simulink model "SteeringWheel"  (R2024b)
settings: configuration reference "STM32H7_Config" (kept outside this file)
settings Model: DataDictionary=Master_Dictionary.sldd  EnableAccessToBaseWorkspace=off  Creator=torni  LastModifiedBy=William
settings ConfigSetRef: SourceName=STM32H7_Config

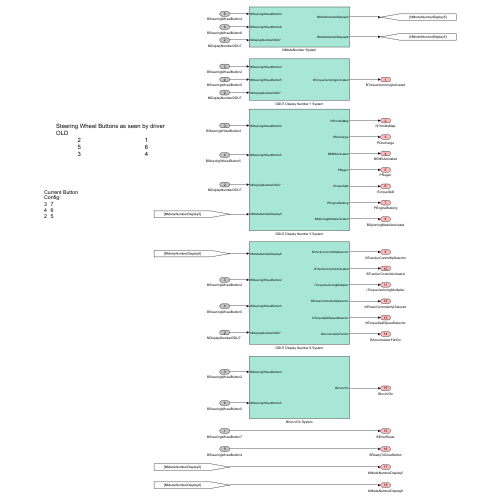
[thumbnail: Simulink's stored preview of the top-level diagram]
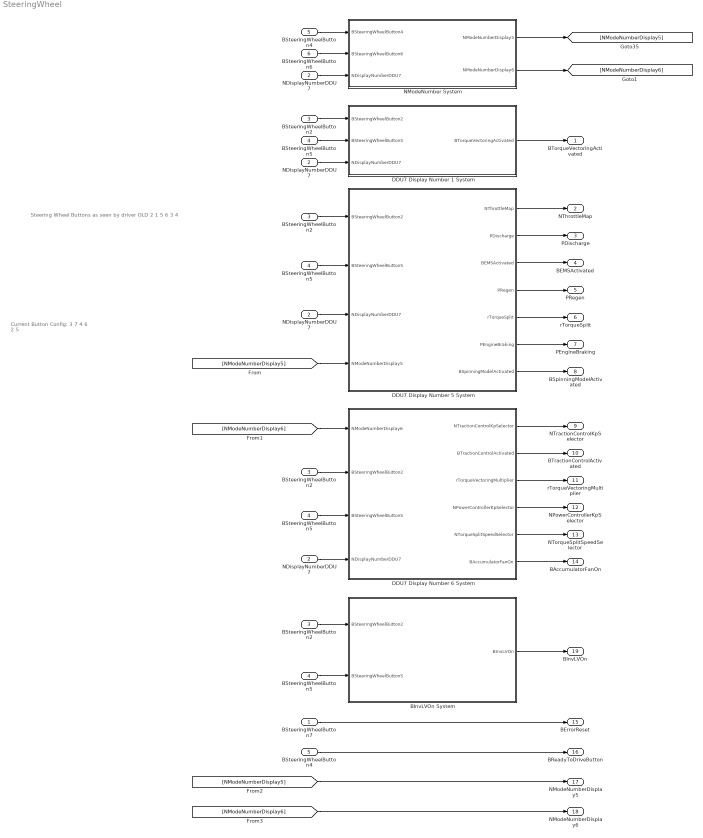
== system SteeringWheel ==
  note: Current Button Config:
      | 3 7
      | 4 6
      | 2 5
  note: Steering Wheel Buttons as seen by driver
      | OLD
      | 2 1
      | 5 6
      | 3 4
  BSteeringWheelButton7 : Inport  OutDataTypeStr=boolean
  NDisplayNumberDDU7 : Inport  Port=2  OutDataTypeStr=double
  "BSteeringWheelButton2 " : Inport  Port=3  OutDataTypeStr=boolean
  "BSteeringWheelButton5 " : Inport  Port=4  OutDataTypeStr=boolean
  BSteeringWheelButton4 : Inport  Port=5  OutDataTypeStr=boolean
  BSteeringWheelButton6 : Inport  Port=6  OutDataTypeStr=boolean
  BInvLVOn System : Subsystem
  "BSteeringWheelButton2 " : InportShadow  Port=3  OutDataTypeStr=boolean
  "BSteeringWheelButton2 " : InportShadow  Port=3  OutDataTypeStr=boolean
  "BSteeringWheelButton2  " : InportShadow  Port=3  OutDataTypeStr=boolean
  "BSteeringWheelButton4 " : InportShadow  Port=5  OutDataTypeStr=boolean
  "BSteeringWheelButton5 " : InportShadow  Port=4  OutDataTypeStr=boolean
  "BSteeringWheelButton5 " : InportShadow  Port=4  OutDataTypeStr=boolean
  "BSteeringWheelButton5   " : InportShadow  Port=4  OutDataTypeStr=boolean
  DDU7 Display Number 1 System : Subsystem
  DDU7 Display Number 5 System : Subsystem
  DDU7 Display Number 6 System : Subsystem
  "NDisplayNumberDDU7 " : InportShadow  Port=2  OutDataTypeStr=double
  "NDisplayNumberDDU7 " : InportShadow  Port=2  OutDataTypeStr=double
  "NDisplayNumberDDU7  " : InportShadow  Port=2  OutDataTypeStr=double
  NModeNumber System : Subsystem
  BTorqueVectoringActivated : Outport  OutDataTypeStr=boolean  VectorParamsAs1DForOutWhenUnconnected=off
  NThrottleMap : Outport  Port=2  OutDataTypeStr=double  VectorParamsAs1DForOutWhenUnconnected=off
  PDischarge : Outport  Port=3  OutDataTypeStr=double  VectorParamsAs1DForOutWhenUnconnected=off
  BEMSActivated : Outport  Port=4  OutDataTypeStr=boolean  VectorParamsAs1DForOutWhenUnconnected=off
  PRegen : Outport  Port=5  OutDataTypeStr=double  VectorParamsAs1DForOutWhenUnconnected=off
  rTorqueSplit : Outport  Port=6  OutDataTypeStr=double  VectorParamsAs1DForOutWhenUnconnected=off
  PEngineBraking : Outport  Port=7  OutDataTypeStr=double  VectorParamsAs1DForOutWhenUnconnected=off
  BSpinningModelActivated : Outport  Port=8  OutDataTypeStr=boolean  VectorParamsAs1DForOutWhenUnconnected=off
  NTractionControlKpSelector : Outport  Port=9  OutDataTypeStr=double  VectorParamsAs1DForOutWhenUnconnected=off
  BTractionControlActivated : Outport  Port=10  OutDataTypeStr=boolean  VectorParamsAs1DForOutWhenUnconnected=off
  rTorqueVectoringMultiplier : Outport  Port=11  OutDataTypeStr=double  VectorParamsAs1DForOutWhenUnconnected=off
  NPowerControllerKpSelector : Outport  Port=12  OutDataTypeStr=double  VectorParamsAs1DForOutWhenUnconnected=off
  NTorqueSplitSpeedSelector : Outport  Port=13  OutDataTypeStr=double  VectorParamsAs1DForOutWhenUnconnected=off
  BAccumulatorFanOn : Outport  Port=14  OutDataTypeStr=boolean  VectorParamsAs1DForOutWhenUnconnected=off
  BErrorReset : Outport  Port=15  OutDataTypeStr=boolean  VectorParamsAs1DForOutWhenUnconnected=off
  BReadyToDriveButton : Outport  Port=16  OutDataTypeStr=boolean  VectorParamsAs1DForOutWhenUnconnected=off
  NModeNumberDisplay5 : Outport  Port=17  OutDataTypeStr=double  VectorParamsAs1DForOutWhenUnconnected=off
  NModeNumberDisplay6 : Outport  Port=18  OutDataTypeStr=double  VectorParamsAs1DForOutWhenUnconnected=off
  BInvLVOn : Outport  Port=19  OutDataTypeStr=boolean  VectorParamsAs1DForOutWhenUnconnected=off
  wires:
  "BSteeringWheelButton5 "/1 -> DDU7 Display Number 1 System/2("BSteeringWheelButton5 ")
  "BSteeringWheelButton2 "/1 -> DDU7 Display Number 1 System/1("BSteeringWheelButton2 ")
  NDisplayNumberDDU7/1 -> DDU7 Display Number 1 System/3(NDisplayNumberDDU7)
  "NDisplayNumberDDU7 "/1 -> DDU7 Display Number 5 System/3(NDisplayNumberDDU7)
  "NDisplayNumberDDU7  "/1 -> DDU7 Display Number 6 System/4("NDisplayNumberDDU7  ")
  NModeNumber System/1(NModeNumberDisplay5) -> [NModeNumberDisplay5]
  NModeNumber System/2(NModeNumberDisplay6) -> [NModeNumberDisplay6]
  "BSteeringWheelButton2  "/1 -> DDU7 Display Number 5 System/1("BSteeringWheelButton2  ")
  "BSteeringWheelButton5   "/1 -> DDU7 Display Number 5 System/2("BSteeringWheelButton5  ")
  "BSteeringWheelButton2 "/1 -> DDU7 Display Number 6 System/2("BSteeringWheelButton2 ")
  "BSteeringWheelButton5 "/1 -> DDU7 Display Number 6 System/3("BSteeringWheelButton5 ")
  DDU7 Display Number 5 System/6(PEngineBraking) -> PEngineBraking/1
  DDU7 Display Number 5 System/1(NThrottleMap) -> NThrottleMap/1
  DDU7 Display Number 5 System/5(rTorqueSplit) -> rTorqueSplit/1
  DDU7 Display Number 5 System/4(PRegen) -> PRegen/1
  DDU7 Display Number 6 System/1(NTractionControlKpSelector) -> NTractionControlKpSelector/1
  DDU7 Display Number 6 System/3(rTorqueVectoringMultiplier) -> rTorqueVectoringMultiplier/1
  DDU7 Display Number 6 System/4(NPowerControllerKpSelector) -> NPowerControllerKpSelector/1
  DDU7 Display Number 6 System/5(NTorqueSplitSpeedSelector) -> NTorqueSplitSpeedSelector/1
  BSteeringWheelButton7/1 -> BErrorReset/1
  "NDisplayNumberDDU7 "/1 -> NModeNumber System/3("NDisplayNumberDDU7 ")
  BSteeringWheelButton4/1 -> NModeNumber System/1("BSteeringWheelButton4 ")
  BSteeringWheelButton6/1 -> NModeNumber System/2("BSteeringWheelButton6 ")
  DDU7 Display Number 5 System/2(PDischarge) -> PDischarge/1
  "BSteeringWheelButton4 "/1 -> BReadyToDriveButton/1
  [NModeNumberDisplay5] -> DDU7 Display Number 5 System/4(NModeNumberDisplay5)
  [NModeNumberDisplay6] -> DDU7 Display Number 6 System/1(NModeNumberDisplay6)
  [NModeNumberDisplay5] -> NModeNumberDisplay5/1
  [NModeNumberDisplay6] -> NModeNumberDisplay6/1
  DDU7 Display Number 6 System/6(BAccumulatorFanOn) -> BAccumulatorFanOn/1
  DDU7 Display Number 6 System/2(BTractionControlActivated) -> BTractionControlActivated/1
  DDU7 Display Number 5 System/7(BSpinningModelActivated) -> BSpinningModelActivated/1
  DDU7 Display Number 5 System/3(BEMSActivated) -> BEMSActivated/1
  DDU7 Display Number 1 System/1(BTorqueVectoringActivated) -> BTorqueVectoringActivated/1
  "BSteeringWheelButton5 "/1 -> BInvLVOn System/2(BSteeringWheelButton5)
  "BSteeringWheelButton2 "/1 -> BInvLVOn System/1("BSteeringWheelButton2 ")
  BInvLVOn System/1(BInvLVOn) -> BInvLVOn/1

== system SteeringWheel/BInvLVOn System ==
  "BSteeringWheelButton2 " : Inport  OutDataTypeStr=boolean
  BSteeringWheelButton5 : Inport  Port=2  OutDataTypeStr=boolean
  AND : Logic  Operator=NAND  AllPortsSameDT=off  OutDataTypeStr=boolean
  BInvLVOn : Outport  OutDataTypeStr=boolean  VectorParamsAs1DForOutWhenUnconnected=off
  wires:
  "BSteeringWheelButton2 "/1 -> AND/1
  BSteeringWheelButton5/1 -> AND/2
  AND/1 -> BInvLVOn/1

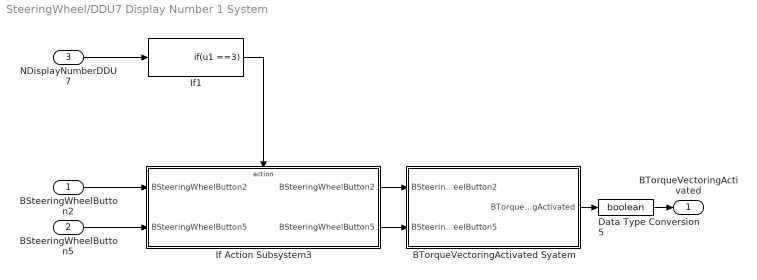
== system SteeringWheel/DDU7 Display Number 1 System ==
  "BSteeringWheelButton2 " : Inport  OutDataTypeStr=boolean
  "BSteeringWheelButton5 " : Inport  Port=2  OutDataTypeStr=boolean
  NDisplayNumberDDU7 : Inport  Port=3  OutDataTypeStr=double
  BTorqueVectoringActivated Syatem : Stateflow chart  TreatAsAtomicUnit=on
  Data Type Conversion5 : DataTypeConversion  OutDataTypeStr=boolean  SaturateOnIntegerOverflow=off  RndMeth=Floor
  If Action Subsystem3 : Subsystem  TreatAsAtomicUnit=on
  If1 : If  IfExpression=u1 ==3  ShowElse=off
  BTorqueVectoringActivated : Outport  OutDataTypeStr=boolean  VectorParamsAs1DForOutWhenUnconnected=off
  wires:
  If Action Subsystem3/1(BSteeringWheelButton2) -> BTorqueVectoringActivated Syatem/1(BSteeringWheelButton2)
  If Action Subsystem3/2(BSteeringWheelButton5) -> BTorqueVectoringActivated Syatem/2(BSteeringWheelButton5)
  If1/1 -> If Action Subsystem3/Action
  NDisplayNumberDDU7/1 -> If1/1
  "BSteeringWheelButton2 "/1 -> If Action Subsystem3/1("BSteeringWheelButton2 ")
  "BSteeringWheelButton5 "/1 -> If Action Subsystem3/2("BSteeringWheelButton5 ")
  Data Type Conversion5/1 -> BTorqueVectoringActivated/1
  BTorqueVectoringActivated Syatem/1(BTorqueVectoringActivated) -> Data Type Conversion5/1

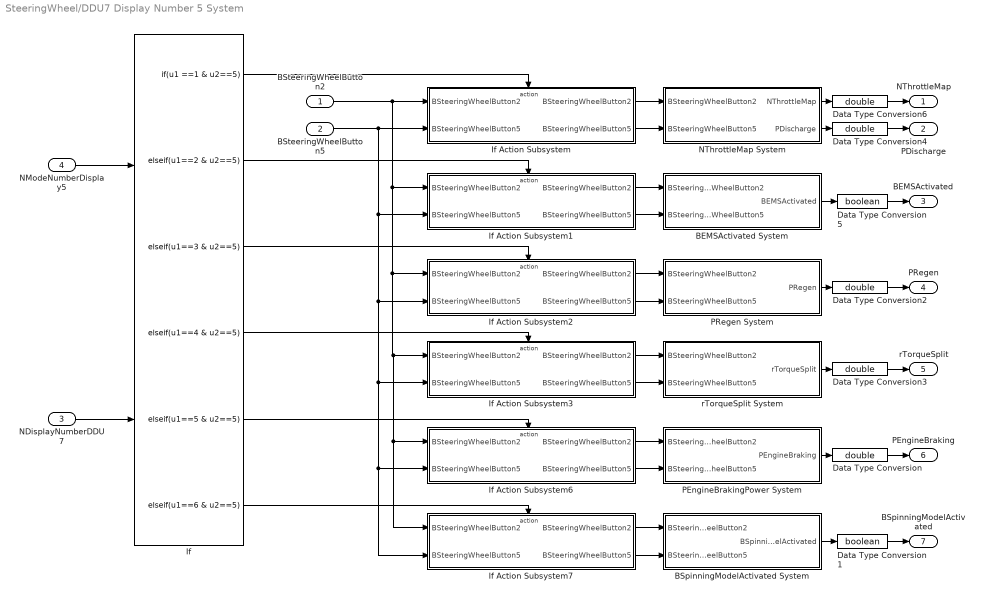
== system SteeringWheel/DDU7 Display Number 5 System ==
  "BSteeringWheelButton2  " : Inport  OutDataTypeStr=boolean
  "BSteeringWheelButton5  " : Inport  Port=2  OutDataTypeStr=boolean
  NDisplayNumberDDU7 : Inport  Port=3  OutDataTypeStr=double
  NModeNumberDisplay5 : Inport  Port=4  OutDataTypeStr=double
  BEMSActivated System : Stateflow chart  TreatAsAtomicUnit=on
  BSpinningModelActivated System : Stateflow chart  TreatAsAtomicUnit=on
  Data Type Conversion{,2..4,6} (5 alike) : DataTypeConversion  OutDataTypeStr=double  SaturateOnIntegerOverflow=off  RndMeth=Floor
  Data Type Conversion1 : DataTypeConversion  OutDataTypeStr=boolean  SaturateOnIntegerOverflow=off  RndMeth=Floor
  Data Type Conversion5 : DataTypeConversion  OutDataTypeStr=boolean  SaturateOnIntegerOverflow=off  RndMeth=Floor
  If : If  NumInputs=2  IfExpression=u1 ==1 & u2==5  ElseIfExpressions=u1==2 & u2==5,u1==3 & u2==5,u1==4 & u2==5 ,u1==5 & u2==5,u1==6 & u2==5  ShowElse=off
  If Action Subsystem : Subsystem  TreatAsAtomicUnit=on
  If Action Subsystem1 : Subsystem  TreatAsAtomicUnit=on
  If Action Subsystem2 : Subsystem  TreatAsAtomicUnit=on
  If Action Subsystem3 : Subsystem  TreatAsAtomicUnit=on
  If Action Subsystem6 : Subsystem  TreatAsAtomicUnit=on
  If Action Subsystem7 : Subsystem  TreatAsAtomicUnit=on
  NThrottleMap System : Stateflow chart  TreatAsAtomicUnit=on
  PEngineBrakingPower System : Stateflow chart  TreatAsAtomicUnit=on
  PRegen System : Stateflow chart  TreatAsAtomicUnit=on
  rTorqueSplit System : Stateflow chart  TreatAsAtomicUnit=on
  NThrottleMap : Outport  OutDataTypeStr=double  VectorParamsAs1DForOutWhenUnconnected=off
  PDischarge : Outport  Port=2  OutDataTypeStr=double  VectorParamsAs1DForOutWhenUnconnected=off
  BEMSActivated : Outport  Port=3  OutDataTypeStr=boolean  VectorParamsAs1DForOutWhenUnconnected=off
  PRegen : Outport  Port=4  OutDataTypeStr=double  VectorParamsAs1DForOutWhenUnconnected=off
  rTorqueSplit : Outport  Port=5  OutDataTypeStr=double  VectorParamsAs1DForOutWhenUnconnected=off
  PEngineBraking : Outport  Port=6  OutDataTypeStr=double  VectorParamsAs1DForOutWhenUnconnected=off
  BSpinningModelActivated : Outport  Port=7  OutDataTypeStr=boolean  VectorParamsAs1DForOutWhenUnconnected=off
  wires:
  NModeNumberDisplay5/1 -> If/1
  If Action Subsystem/2(BSteeringWheelButton5) -> NThrottleMap System/2(BSteeringWheelButton5)
  If Action Subsystem/1(BSteeringWheelButton2) -> NThrottleMap System/1(BSteeringWheelButton2)
  NThrottleMap System/1(NThrottleMap) -> Data Type Conversion6/1
  BEMSActivated System/1(BEMSActivated) -> Data Type Conversion5/1
  If Action Subsystem2/1(BSteeringWheelButton2) -> PRegen System/1(BSteeringWheelButton2)
  If Action Subsystem2/2(BSteeringWheelButton5) -> PRegen System/2(BSteeringWheelButton5)
  PRegen System/1(PRegen) -> Data Type Conversion2/1
  If Action Subsystem3/1(BSteeringWheelButton2) -> rTorqueSplit System/1(BSteeringWheelButton2)
  If Action Subsystem3/2(BSteeringWheelButton5) -> rTorqueSplit System/2(BSteeringWheelButton5)
  rTorqueSplit System/1(rTorqueSplit) -> Data Type Conversion3/1
  If Action Subsystem6/2(BSteeringWheelButton5) -> PEngineBrakingPower System/2(BSteeringWheelButton5)
  PEngineBrakingPower System/1(PEngineBraking) -> Data Type Conversion/1
  If Action Subsystem6/1(BSteeringWheelButton2) -> PEngineBrakingPower System/1(BSteeringWheelButton2)
  If Action Subsystem7/2(BSteeringWheelButton5) -> BSpinningModelActivated System/2(BSteeringWheelButton5)
  BSpinningModelActivated System/1(BSpinningModelActivated) -> Data Type Conversion1/1
  If Action Subsystem7/1(BSteeringWheelButton2) -> BSpinningModelActivated System/1(BSteeringWheelButton2)
  If/4 -> If Action Subsystem3/Action
  If/3 -> If Action Subsystem2/Action
  If/2 -> If Action Subsystem1/Action
  If/1 -> If Action Subsystem/Action
  If/5 -> If Action Subsystem6/Action
  If/6 -> If Action Subsystem7/Action
  NDisplayNumberDDU7/1 -> If/2
  "BSteeringWheelButton5  "/1 -> If Action Subsystem6/2("BSteeringWheelButton5  "), If Action Subsystem7/2("BSteeringWheelButton5  "), If Action Subsystem3/2("BSteeringWheelButton5  "), If Action Subsystem2/2("BSteeringWheelButton5  "), If Action Subsystem1/2("BSteeringWheelButton5  "), If Action Subsystem/2("BSteeringWheelButton5  ")
  "BSteeringWheelButton2  "/1 -> If Action Subsystem6/1("BSteeringWheelButton2  "), If Action Subsystem7/1("BSteeringWheelButton2  "), If Action Subsystem3/1("BSteeringWheelButton2  "), If Action Subsystem2/1("BSteeringWheelButton2  "), If Action Subsystem1/1("BSteeringWheelButton2  "), If Action Subsystem/1("BSteeringWheelButton2  ")
  If Action Subsystem1/1(BSteeringWheelButton2) -> BEMSActivated System/1(BSteeringWheelButton2)
  If Action Subsystem1/2(BSteeringWheelButton5) -> BEMSActivated System/2(BSteeringWheelButton5)
  NThrottleMap System/2(PDischarge) -> Data Type Conversion4/1
  Data Type Conversion5/1 -> BEMSActivated/1
  Data Type Conversion1/1 -> BSpinningModelActivated/1
  Data Type Conversion/1 -> PEngineBraking/1
  Data Type Conversion2/1 -> PRegen/1
  Data Type Conversion3/1 -> rTorqueSplit/1
  Data Type Conversion4/1 -> PDischarge/1
  Data Type Conversion6/1 -> NThrottleMap/1

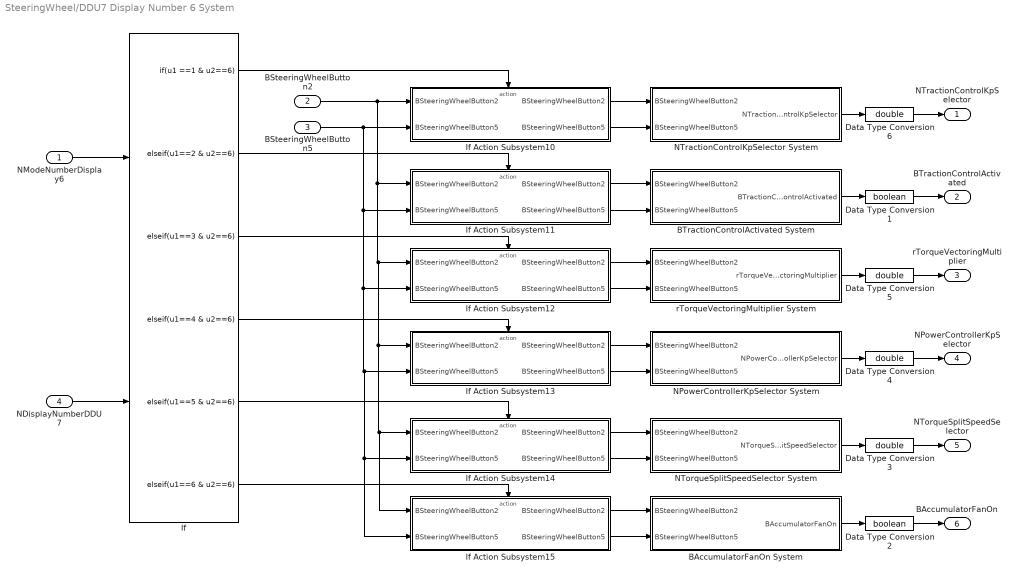
== system SteeringWheel/DDU7 Display Number 6 System ==
  NModeNumberDisplay6 : Inport  OutDataTypeStr=double
  "BSteeringWheelButton2 " : Inport  Port=2  OutDataTypeStr=boolean
  "BSteeringWheelButton5 " : Inport  Port=3  OutDataTypeStr=boolean
  "NDisplayNumberDDU7  " : Inport  Port=4  OutDataTypeStr=double
  BAccumulatorFanOn System : Stateflow chart  TreatAsAtomicUnit=on
  BTractionControlActivated System : Stateflow chart  TreatAsAtomicUnit=on
  Data Type Conversion1 : DataTypeConversion  OutDataTypeStr=boolean  SaturateOnIntegerOverflow=off  RndMeth=Floor
  Data Type Conversion2 : DataTypeConversion  OutDataTypeStr=boolean  SaturateOnIntegerOverflow=off  RndMeth=Floor
  Data Type Conversion{3..6} (4 alike) : DataTypeConversion  OutDataTypeStr=double  SaturateOnIntegerOverflow=off  RndMeth=Floor
  If : If  NumInputs=2  IfExpression=u1 ==1 & u2==6  ElseIfExpressions=u1==2 & u2==6,u1==3 & u2==6,u1==4 & u2==6,u1==5 & u2==6,u1==6 & u2==6  ShowElse=off
  If Action Subsystem10 : Subsystem  TreatAsAtomicUnit=on
  If Action Subsystem11 : Subsystem  TreatAsAtomicUnit=on
  If Action Subsystem12 : Subsystem  TreatAsAtomicUnit=on
  If Action Subsystem13 : Subsystem  TreatAsAtomicUnit=on
  If Action Subsystem14 : Subsystem  TreatAsAtomicUnit=on
  If Action Subsystem15 : Subsystem  TreatAsAtomicUnit=on
  NPowerControllerKpSelector System : Stateflow chart  TreatAsAtomicUnit=on
  NTorqueSplitSpeedSelector System : Stateflow chart  TreatAsAtomicUnit=on
  NTractionControlKpSelector System : Stateflow chart  TreatAsAtomicUnit=on
  rTorqueVectoringMultiplier System : Stateflow chart  TreatAsAtomicUnit=on
  NTractionControlKpSelector : Outport  OutDataTypeStr=double  VectorParamsAs1DForOutWhenUnconnected=off
  BTractionControlActivated : Outport  Port=2  OutDataTypeStr=boolean  VectorParamsAs1DForOutWhenUnconnected=off
  rTorqueVectoringMultiplier : Outport  Port=3  OutDataTypeStr=double  VectorParamsAs1DForOutWhenUnconnected=off
  NPowerControllerKpSelector : Outport  Port=4  OutDataTypeStr=double  VectorParamsAs1DForOutWhenUnconnected=off
  NTorqueSplitSpeedSelector : Outport  Port=5  OutDataTypeStr=double  VectorParamsAs1DForOutWhenUnconnected=off
  BAccumulatorFanOn : Outport  Port=6  OutDataTypeStr=boolean  VectorParamsAs1DForOutWhenUnconnected=off
  wires:
  If Action Subsystem15/1(BSteeringWheelButton2) -> BAccumulatorFanOn System/1(BSteeringWheelButton2)
  BAccumulatorFanOn System/1(BAccumulatorFanOn) -> Data Type Conversion2/1
  If Action Subsystem15/2(BSteeringWheelButton5) -> BAccumulatorFanOn System/2(BSteeringWheelButton5)
  If Action Subsystem14/1(BSteeringWheelButton2) -> NTorqueSplitSpeedSelector System/1(BSteeringWheelButton2)
  NTorqueSplitSpeedSelector System/1(NTorqueSplitSpeedSelector) -> Data Type Conversion3/1
  If Action Subsystem14/2(BSteeringWheelButton5) -> NTorqueSplitSpeedSelector System/2(BSteeringWheelButton5)
  If Action Subsystem13/2(BSteeringWheelButton5) -> NPowerControllerKpSelector System/2(BSteeringWheelButton5)
  If Action Subsystem13/1(BSteeringWheelButton2) -> NPowerControllerKpSelector System/1(BSteeringWheelButton2)
  NPowerControllerKpSelector System/1(NPowerControllerKpSelector) -> Data Type Conversion4/1
  rTorqueVectoringMultiplier System/1(rTorqueVectoringMultiplier) -> Data Type Conversion5/1
  If Action Subsystem12/2(BSteeringWheelButton5) -> rTorqueVectoringMultiplier System/2(BSteeringWheelButton5)
  If Action Subsystem12/1(BSteeringWheelButton2) -> rTorqueVectoringMultiplier System/1(BSteeringWheelButton2)
  BTractionControlActivated System/1(BTractionControlActivated) -> Data Type Conversion1/1
  If Action Subsystem11/2(BSteeringWheelButton5) -> BTractionControlActivated System/2(BSteeringWheelButton5)
  If Action Subsystem11/1(BSteeringWheelButton2) -> BTractionControlActivated System/1(BSteeringWheelButton2)
  NTractionControlKpSelector System/1(NTractionControlKpSelector) -> Data Type Conversion6/1
  "BSteeringWheelButton5 "/1 -> If Action Subsystem15/2("BSteeringWheelButton5  "), If Action Subsystem14/2("BSteeringWheelButton5  "), If Action Subsystem13/2("BSteeringWheelButton5  "), If Action Subsystem12/2("BSteeringWheelButton5  "), If Action Subsystem11/2("BSteeringWheelButton5  "), If Action Subsystem10/2("BSteeringWheelButton5  ")
  If/2 -> If Action Subsystem11/Action
  If/6 -> If Action Subsystem15/Action
  If/4 -> If Action Subsystem13/Action
  If/3 -> If Action Subsystem12/Action
  If/1 -> If Action Subsystem10/Action
  "BSteeringWheelButton2 "/1 -> If Action Subsystem15/1("BSteeringWheelButton2  "), If Action Subsystem14/1("BSteeringWheelButton2  "), If Action Subsystem13/1("BSteeringWheelButton2  "), If Action Subsystem12/1("BSteeringWheelButton2  "), If Action Subsystem11/1("BSteeringWheelButton2  "), If Action Subsystem10/1("BSteeringWheelButton2  ")
  "NDisplayNumberDDU7  "/1 -> If/2
  NModeNumberDisplay6/1 -> If/1
  If/5 -> If Action Subsystem14/Action
  If Action Subsystem10/1(BSteeringWheelButton2) -> NTractionControlKpSelector System/1(BSteeringWheelButton2)
  If Action Subsystem10/2(BSteeringWheelButton5) -> NTractionControlKpSelector System/2(BSteeringWheelButton5)
  Data Type Conversion2/1 -> BAccumulatorFanOn/1
  Data Type Conversion1/1 -> BTractionControlActivated/1
  Data Type Conversion3/1 -> NTorqueSplitSpeedSelector/1
  Data Type Conversion4/1 -> NPowerControllerKpSelector/1
  Data Type Conversion5/1 -> rTorqueVectoringMultiplier/1
  Data Type Conversion6/1 -> NTractionControlKpSelector/1

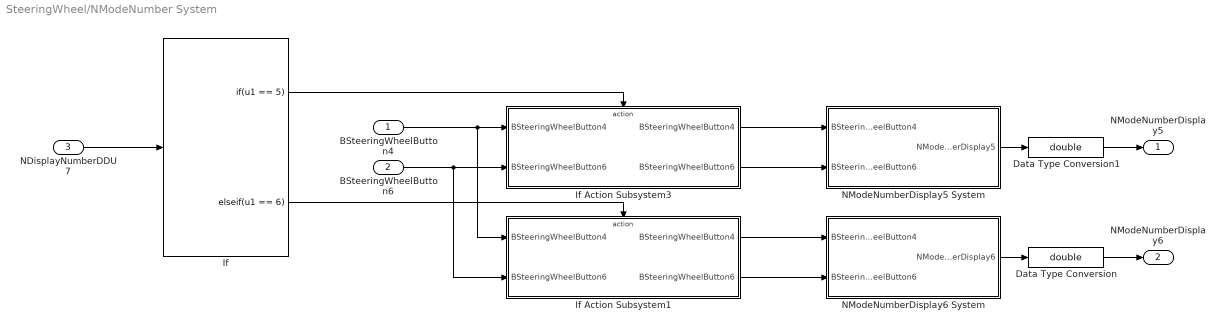
== system SteeringWheel/NModeNumber System ==
  "BSteeringWheelButton4 " : Inport  OutDataTypeStr=boolean
  "BSteeringWheelButton6 " : Inport  Port=2  OutDataTypeStr=boolean
  "NDisplayNumberDDU7 " : Inport  Port=3  OutDataTypeStr=double
  Data Type Conversion : DataTypeConversion  OutDataTypeStr=double  SaturateOnIntegerOverflow=off  RndMeth=Floor
  Data Type Conversion1 : DataTypeConversion  OutDataTypeStr=double  SaturateOnIntegerOverflow=off  RndMeth=Floor
  If : If  IfExpression=u1 == 5  ElseIfExpressions=u1 == 6  ShowElse=off
  If Action Subsystem1 : Subsystem  TreatAsAtomicUnit=on
  If Action Subsystem3 : Subsystem  TreatAsAtomicUnit=on
  NModeNumberDisplay5 System : Stateflow chart  TreatAsAtomicUnit=on
  NModeNumberDisplay6 System : Stateflow chart  TreatAsAtomicUnit=on
  NModeNumberDisplay5 : Outport  OutDataTypeStr=double  VectorParamsAs1DForOutWhenUnconnected=off
  NModeNumberDisplay6 : Outport  Port=2  OutDataTypeStr=double  VectorParamsAs1DForOutWhenUnconnected=off
  wires:
  NModeNumberDisplay5 System/1(NModeNumberDisplay5) -> Data Type Conversion1/1
  If Action Subsystem3/1(BSteeringWheelButton4) -> NModeNumberDisplay5 System/1(BSteeringWheelButton4)
  If Action Subsystem3/2(BSteeringWheelButton6) -> NModeNumberDisplay5 System/2(BSteeringWheelButton6)
  NModeNumberDisplay6 System/1(NModeNumberDisplay6) -> Data Type Conversion/1
  If Action Subsystem1/1(BSteeringWheelButton4) -> NModeNumberDisplay6 System/1(BSteeringWheelButton4)
  If Action Subsystem1/2(BSteeringWheelButton6) -> NModeNumberDisplay6 System/2(BSteeringWheelButton6)
  "NDisplayNumberDDU7 "/1 -> If/1
  "BSteeringWheelButton6 "/1 -> If Action Subsystem1/2("BSteeringWheelButton6 "), If Action Subsystem3/2("BSteeringWheelButton6 ")
  "BSteeringWheelButton4 "/1 -> If Action Subsystem1/1("BSteeringWheelButton4 "), If Action Subsystem3/1("BSteeringWheelButton4 ")
  If/1 -> If Action Subsystem3/Action
  If/2 -> If Action Subsystem1/Action
  Data Type Conversion1/1 -> NModeNumberDisplay5/1
  Data Type Conversion/1 -> NModeNumberDisplay6/1

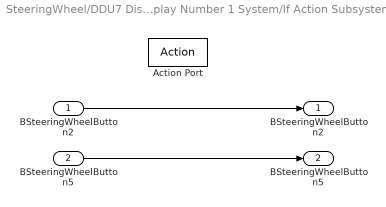
== system SteeringWheel/DDU7 Display Number 1 System/If Action Subsystem3 ==
  "BSteeringWheelButton2 " : Inport  OutDataTypeStr=boolean
  "BSteeringWheelButton5 " : Inport  Port=2  OutDataTypeStr=boolean
  Action Port : ActionPort  ActionPortLabel=if { }
  BSteeringWheelButton2 : Outport  OutDataTypeStr=boolean  VectorParamsAs1DForOutWhenUnconnected=off
  BSteeringWheelButton5 : Outport  Port=2  OutDataTypeStr=boolean  VectorParamsAs1DForOutWhenUnconnected=off
  wires:
  "BSteeringWheelButton2 "/1 -> BSteeringWheelButton2/1
  "BSteeringWheelButton5 "/1 -> BSteeringWheelButton5/1

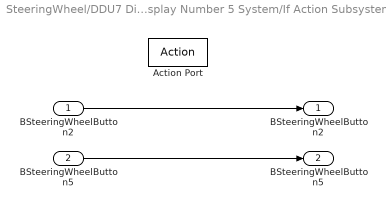
== system SteeringWheel/DDU7 Display Number 5 System/If Action Subsystem ==
  "BSteeringWheelButton2  " : Inport  OutDataTypeStr=boolean
  "BSteeringWheelButton5  " : Inport  Port=2  OutDataTypeStr=boolean
  Action Port : ActionPort  ActionPortLabel=if { }
  BSteeringWheelButton2 : Outport  OutDataTypeStr=boolean  VectorParamsAs1DForOutWhenUnconnected=off
  BSteeringWheelButton5 : Outport  Port=2  OutDataTypeStr=boolean  VectorParamsAs1DForOutWhenUnconnected=off
  wires:
  "BSteeringWheelButton2  "/1 -> BSteeringWheelButton2/1
  "BSteeringWheelButton5  "/1 -> BSteeringWheelButton5/1

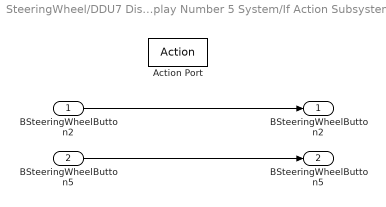
== system SteeringWheel/DDU7 Display Number 5 System/If Action Subsystem1 ==
  "BSteeringWheelButton2  " : Inport  OutDataTypeStr=boolean
  "BSteeringWheelButton5  " : Inport  Port=2  OutDataTypeStr=boolean
  Action Port : ActionPort  ActionPortLabel=elseif { }
  BSteeringWheelButton2 : Outport  OutDataTypeStr=boolean  VectorParamsAs1DForOutWhenUnconnected=off
  BSteeringWheelButton5 : Outport  Port=2  OutDataTypeStr=boolean  VectorParamsAs1DForOutWhenUnconnected=off
  wires:
  "BSteeringWheelButton5  "/1 -> BSteeringWheelButton5/1
  "BSteeringWheelButton2  "/1 -> BSteeringWheelButton2/1

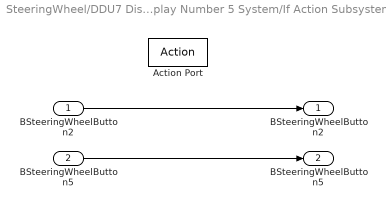
== system SteeringWheel/DDU7 Display Number 5 System/If Action Subsystem2 ==
  "BSteeringWheelButton2  " : Inport  OutDataTypeStr=boolean
  "BSteeringWheelButton5  " : Inport  Port=2  OutDataTypeStr=boolean
  Action Port : ActionPort  ActionPortLabel=elseif { }
  BSteeringWheelButton2 : Outport  OutDataTypeStr=boolean  VectorParamsAs1DForOutWhenUnconnected=off
  BSteeringWheelButton5 : Outport  Port=2  OutDataTypeStr=boolean  VectorParamsAs1DForOutWhenUnconnected=off
  wires:
  "BSteeringWheelButton2  "/1 -> BSteeringWheelButton2/1
  "BSteeringWheelButton5  "/1 -> BSteeringWheelButton5/1

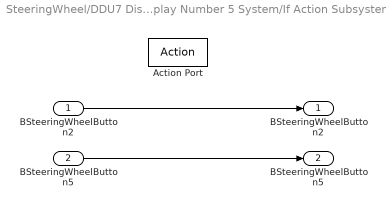
== system SteeringWheel/DDU7 Display Number 5 System/If Action Subsystem3 ==
  "BSteeringWheelButton2  " : Inport  OutDataTypeStr=boolean
  "BSteeringWheelButton5  " : Inport  Port=2  OutDataTypeStr=boolean
  Action Port : ActionPort  ActionPortLabel=elseif { }
  BSteeringWheelButton2 : Outport  OutDataTypeStr=boolean  VectorParamsAs1DForOutWhenUnconnected=off
  BSteeringWheelButton5 : Outport  Port=2  OutDataTypeStr=boolean  VectorParamsAs1DForOutWhenUnconnected=off
  wires:
  "BSteeringWheelButton5  "/1 -> BSteeringWheelButton5/1
  "BSteeringWheelButton2  "/1 -> BSteeringWheelButton2/1

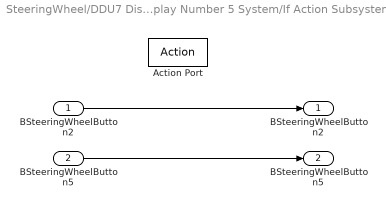
== system SteeringWheel/DDU7 Display Number 5 System/If Action Subsystem6 ==
  "BSteeringWheelButton2  " : Inport  OutDataTypeStr=boolean
  "BSteeringWheelButton5  " : Inport  Port=2  OutDataTypeStr=boolean
  Action Port : ActionPort  ActionPortLabel=elseif { }
  BSteeringWheelButton2 : Outport  OutDataTypeStr=boolean  VectorParamsAs1DForOutWhenUnconnected=off
  BSteeringWheelButton5 : Outport  Port=2  OutDataTypeStr=boolean  VectorParamsAs1DForOutWhenUnconnected=off
  wires:
  "BSteeringWheelButton2  "/1 -> BSteeringWheelButton2/1
  "BSteeringWheelButton5  "/1 -> BSteeringWheelButton5/1

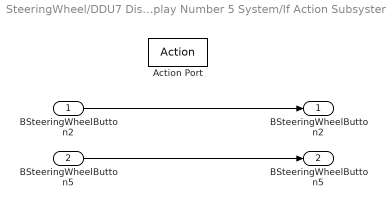
== system SteeringWheel/DDU7 Display Number 5 System/If Action Subsystem7 ==
  "BSteeringWheelButton2  " : Inport  OutDataTypeStr=boolean
  "BSteeringWheelButton5  " : Inport  Port=2  OutDataTypeStr=boolean
  Action Port : ActionPort  ActionPortLabel=elseif { }
  BSteeringWheelButton2 : Outport  OutDataTypeStr=boolean  VectorParamsAs1DForOutWhenUnconnected=off
  BSteeringWheelButton5 : Outport  Port=2  OutDataTypeStr=boolean  VectorParamsAs1DForOutWhenUnconnected=off
  wires:
  "BSteeringWheelButton5  "/1 -> BSteeringWheelButton5/1
  "BSteeringWheelButton2  "/1 -> BSteeringWheelButton2/1

== system SteeringWheel/DDU7 Display Number 6 System/If Action Subsystem10 ==
  "BSteeringWheelButton2  " : Inport  OutDataTypeStr=boolean
  "BSteeringWheelButton5  " : Inport  Port=2  OutDataTypeStr=boolean
  Action Port : ActionPort  ActionPortLabel=if { }
  BSteeringWheelButton2 : Outport  OutDataTypeStr=boolean  VectorParamsAs1DForOutWhenUnconnected=off
  BSteeringWheelButton5 : Outport  Port=2  OutDataTypeStr=boolean  VectorParamsAs1DForOutWhenUnconnected=off
  wires:
  "BSteeringWheelButton5  "/1 -> BSteeringWheelButton5/1
  "BSteeringWheelButton2  "/1 -> BSteeringWheelButton2/1

== system SteeringWheel/DDU7 Display Number 6 System/If Action Subsystem11 ==
  "BSteeringWheelButton2  " : Inport  OutDataTypeStr=boolean
  "BSteeringWheelButton5  " : Inport  Port=2  OutDataTypeStr=boolean
  Action Port : ActionPort  ActionPortLabel=elseif { }
  BSteeringWheelButton2 : Outport  OutDataTypeStr=boolean  VectorParamsAs1DForOutWhenUnconnected=off
  BSteeringWheelButton5 : Outport  Port=2  OutDataTypeStr=boolean  VectorParamsAs1DForOutWhenUnconnected=off
  wires:
  "BSteeringWheelButton2  "/1 -> BSteeringWheelButton2/1
  "BSteeringWheelButton5  "/1 -> BSteeringWheelButton5/1

== system SteeringWheel/DDU7 Display Number 6 System/If Action Subsystem12 ==
  "BSteeringWheelButton2  " : Inport  OutDataTypeStr=boolean
  "BSteeringWheelButton5  " : Inport  Port=2  OutDataTypeStr=boolean
  Action Port : ActionPort  ActionPortLabel=elseif { }
  BSteeringWheelButton2 : Outport  OutDataTypeStr=boolean  VectorParamsAs1DForOutWhenUnconnected=off
  BSteeringWheelButton5 : Outport  Port=2  OutDataTypeStr=boolean  VectorParamsAs1DForOutWhenUnconnected=off
  wires:
  "BSteeringWheelButton5  "/1 -> BSteeringWheelButton5/1
  "BSteeringWheelButton2  "/1 -> BSteeringWheelButton2/1

== system SteeringWheel/DDU7 Display Number 6 System/If Action Subsystem13 ==
  "BSteeringWheelButton2  " : Inport  OutDataTypeStr=boolean
  "BSteeringWheelButton5  " : Inport  Port=2  OutDataTypeStr=boolean
  Action Port : ActionPort  ActionPortLabel=elseif { }
  BSteeringWheelButton2 : Outport  OutDataTypeStr=boolean  VectorParamsAs1DForOutWhenUnconnected=off
  BSteeringWheelButton5 : Outport  Port=2  OutDataTypeStr=boolean  VectorParamsAs1DForOutWhenUnconnected=off
  wires:
  "BSteeringWheelButton2  "/1 -> BSteeringWheelButton2/1
  "BSteeringWheelButton5  "/1 -> BSteeringWheelButton5/1

== system SteeringWheel/DDU7 Display Number 6 System/If Action Subsystem14 ==
  "BSteeringWheelButton2  " : Inport  OutDataTypeStr=boolean
  "BSteeringWheelButton5  " : Inport  Port=2  OutDataTypeStr=boolean
  Action Port : ActionPort  ActionPortLabel=elseif { }
  BSteeringWheelButton2 : Outport  OutDataTypeStr=boolean  VectorParamsAs1DForOutWhenUnconnected=off
  BSteeringWheelButton5 : Outport  Port=2  OutDataTypeStr=boolean  VectorParamsAs1DForOutWhenUnconnected=off
  wires:
  "BSteeringWheelButton5  "/1 -> BSteeringWheelButton5/1
  "BSteeringWheelButton2  "/1 -> BSteeringWheelButton2/1

== system SteeringWheel/DDU7 Display Number 6 System/If Action Subsystem15 ==
  "BSteeringWheelButton2  " : Inport  OutDataTypeStr=boolean
  "BSteeringWheelButton5  " : Inport  Port=2  OutDataTypeStr=boolean
  Action Port : ActionPort  ActionPortLabel=elseif { }
  BSteeringWheelButton2 : Outport  OutDataTypeStr=boolean  VectorParamsAs1DForOutWhenUnconnected=off
  BSteeringWheelButton5 : Outport  Port=2  OutDataTypeStr=boolean  VectorParamsAs1DForOutWhenUnconnected=off
  wires:
  "BSteeringWheelButton2  "/1 -> BSteeringWheelButton2/1
  "BSteeringWheelButton5  "/1 -> BSteeringWheelButton5/1

== system SteeringWheel/NModeNumber System/If Action Subsystem1 ==
  "BSteeringWheelButton4 " : Inport  OutDataTypeStr=boolean
  "BSteeringWheelButton6 " : Inport  Port=2  OutDataTypeStr=boolean
  Action Port : ActionPort  ActionPortLabel=elseif { }
  BSteeringWheelButton4 : Outport  OutDataTypeStr=boolean  VectorParamsAs1DForOutWhenUnconnected=off
  BSteeringWheelButton6 : Outport  Port=2  OutDataTypeStr=boolean  VectorParamsAs1DForOutWhenUnconnected=off
  wires:
  "BSteeringWheelButton6 "/1 -> BSteeringWheelButton6/1
  "BSteeringWheelButton4 "/1 -> BSteeringWheelButton4/1

== system SteeringWheel/NModeNumber System/If Action Subsystem3 ==
  "BSteeringWheelButton4 " : Inport  OutDataTypeStr=boolean
  "BSteeringWheelButton6 " : Inport  Port=2  OutDataTypeStr=boolean
  Action Port : ActionPort  ActionPortLabel=if { }
  BSteeringWheelButton4 : Outport  OutDataTypeStr=boolean  VectorParamsAs1DForOutWhenUnconnected=off
  BSteeringWheelButton6 : Outport  Port=2  OutDataTypeStr=boolean  VectorParamsAs1DForOutWhenUnconnected=off
  wires:
  "BSteeringWheelButton4 "/1 -> BSteeringWheelButton4/1
  "BSteeringWheelButton6 "/1 -> BSteeringWheelButton6/1

== stateflow chart SteeringWheel/DDU7 Display Number 5 System/BEMSActivated System ==
  state Map12
    entry:
    BEMSActivated = 1;
  state Map11
    entry, during:
    BEMSActivated = 0;
  Map11 -> Map12 [order 2] : after(500,tick)
      | [BSteeringWheelButton5 ==1]
  Map12 -> Map11 [order 2] : after(500,tick)
      | [BSteeringWheelButton2 == 1]
  (default) -> Map11
  Map12 -> Map11 [order 1] : after(500,tick)
      | [BSteeringWheelButton5 ==1]
  Map11 -> Map12 [order 1] : after(500,tick)
      | [BSteeringWheelButton2 == 1]
  data: BEMSActivated output double; BSteeringWheelButton2 input boolean; BSteeringWheelButton5 input boolean

== stateflow chart SteeringWheel/DDU7 Display Number 5 System/PEngineBrakingPower System ==
  state Map12
    entry:
    PEngineBraking = 14;
  state Map9
    entry, during:
    PEngineBraking = 6;
  state Map11
    entry, during:
    PEngineBraking = 10;
  state Map7
    entry, during:
    PEngineBraking = 0;
  state Map10
    entry, during:
    PEngineBraking = 8;
  state Map8
    entry, during:
    PEngineBraking = 4;
  Map9 -> Map10 [order 2] : after(500,tick)
      | [BSteeringWheelButton2 == 1]
  Map8 -> Map9 [order 2] : after(500,tick)
      | [BSteeringWheelButton2 == 1]
  Map10 -> Map11 [order 2] : after(500,tick)
      | [BSteeringWheelButton2 == 1]
  Map7 -> Map8 [order 2] : after(500,tick)
      | [BSteeringWheelButton2 == 1]
  (default) -> Map11
  Map12 -> Map7 [order 1] : after(500,tick)
      | [BSteeringWheelButton2 == 1]
  Map12 -> Map11 [order 2] : after(500,tick)
      | [BSteeringWheelButton5 ==1]
  Map11 -> Map12 [order 2] : after(500,tick)
      | [BSteeringWheelButton2 == 1]
  Map7 -> Map12 [order 1] : after(500,tick)
      | [BSteeringWheelButton5 ==1]
  Map8 -> Map7 [order 1] : after(500,tick)
      | [BSteeringWheelButton5 ==1]
  Map9 -> Map8 [order 1] : after(500,tick)
      | [BSteeringWheelButton5 ==1]
  Map10 -> Map9 [order 1] : after(500,tick)
      | [BSteeringWheelButton5 ==1]
  Map11 -> Map10 [order 1] : after(500,tick)
      | [BSteeringWheelButton5 ==1]
  data: PEngineBraking output double; BSteeringWheelButton2 input boolean; BSteeringWheelButton5 input boolean

== stateflow chart SteeringWheel/NModeNumber System/NModeNumberDisplay5 System ==
  state Reset10
    Reset=1;
  state Reset4
    Reset=1;
  state Reset
    Reset=1;
  state Reset1
    Reset=1;
  state Reset2
    Reset=1;
  state Reset3
    Reset=1;
  state Mode12
    entry:
    NModeNumberDisplay5 = 1;
    Reset =0;
  state Mode7
    entry, during:
    NModeNumberDisplay5 = 2;
    Reset =0;
  state Mode8
    entry, during:
    NModeNumberDisplay5 = 3;
    Reset =0;
  state Mode11
    entry, during:
    NModeNumberDisplay5 = 4;
    Reset =0;
  state Mode10
    entry, during:
    NModeNumberDisplay5 = 6;
    Reset =0;
  state Mode9
    entry, during:
    NModeNumberDisplay5 = 5;
    Reset =0;
  state Reset5
    Reset=1;
  state Reset8
    Reset=1;
  state Reset9
    Reset=1;
  state Reset7
    Reset=1;
  state Reset6
    Reset=1;
  state Reset11
    Reset=1;
  Mode10 -> Reset10 [order 2] : after(500,tick)
      | [BSteeringWheelButton4 == 1]
  Reset10 -> Mode12 : after(50,tick)
  Reset4 -> Mode10 : after(50,tick)
  Reset2 -> Mode11 : after(50,tick)
  Reset1 -> Mode8 : after(50,tick)
  Reset3 -> Mode9 : after(50,tick)
  Mode9 -> Reset4 [order 1] : after(500,tick)
      | [BSteeringWheelButton4 == 1]
  Reset -> Mode7 : after(50,tick)
  Mode12 -> Reset [order 1] : after(500,tick)
      | [BSteeringWheelButton4 == 1]
  Mode11 -> Reset3 [order 1] : after(500,tick)
      | [BSteeringWheelButton4 == 1]
  Mode7 -> Reset1 [order 2] : after(500,tick)
      | [BSteeringWheelButton4 == 1]
  Mode8 -> Reset2 [order 2] : after(500,tick)
      | [BSteeringWheelButton4 == 1]
  (default) -> Mode12
  Mode7 -> Reset9 [order 1] : after(500,tick)
      | [BSteeringWheelButton6 ==1]
  Reset8 -> Mode7 : after(50,tick)
  Mode8 -> Reset8 [order 1] : after(500,tick)
      | [BSteeringWheelButton6 ==1]
  Reset7 -> Mode8 : after(50,tick)
  Reset11 -> Mode10 : after(50,tick)
  Mode11 -> Reset7 [order 2] : after(500,tick)
      | [BSteeringWheelButton6 ==1]
  Reset6 -> Mode11 : after(50,tick)
  Mode9 -> Reset6 [order 2] : after(500,tick)
      | [BSteeringWheelButton6 ==1]
  Reset5 -> Mode9 : after(50,tick)
  Mode10 -> Reset5 [order 1] : after(500,tick)
      | [BSteeringWheelButton6 ==1]
  Mode12 -> Reset11 [order 2] : after(500,tick)
      | [BSteeringWheelButton6 ==1]
  Reset9 -> Mode12 : after(50,tick)
  data: BSteeringWheelButton4 input boolean; NModeNumberDisplay5 output; BSteeringWheelButton6 input boolean; Reset local

== stateflow chart SteeringWheel/DDU7 Display Number 5 System/rTorqueSplit System ==
  state Map12
    entry:
    rTorqueSplit = 0.5;
  state Map7
    entry, during:
    rTorqueSplit = 0.6;
  state Map8
    entry, during:
    rTorqueSplit = 0.7;
  state Map9
    entry, during:
    rTorqueSplit = 0.8;
  state Map10
    entry, during:
    rTorqueSplit = 0.9;
  state Map11
    entry, during:
    rTorqueSplit = 1;
  (default) -> Map8
  Map9 -> Map10 [order 2] : after(500,tick)
      | [BSteeringWheelButton2 == 1]
  Map8 -> Map9 [order 2] : after(500,tick)
      | [BSteeringWheelButton2 == 1]
  Map10 -> Map11 [order 2] : after(500,tick)
      | [BSteeringWheelButton2 == 1]
  Map7 -> Map8 [order 2] : after(500,tick)
      | [BSteeringWheelButton2 == 1]
  Map12 -> Map7 [order 1] : after(500,tick)
      | [BSteeringWheelButton2 == 1]
  Map12 -> Map11 [order 2] : after(500,tick)
      | [BSteeringWheelButton5 ==1]
  Map11 -> Map12 [order 2] : after(500,tick)
      | [BSteeringWheelButton2 == 1]
  Map7 -> Map12 [order 1] : after(500,tick)
      | [BSteeringWheelButton5 ==1]
  Map8 -> Map7 [order 1] : after(500,tick)
      | [BSteeringWheelButton5 ==1]
  Map9 -> Map8 [order 1] : after(500,tick)
      | [BSteeringWheelButton5 ==1]
  Map10 -> Map9 [order 1] : after(500,tick)
      | [BSteeringWheelButton5 ==1]
  Map11 -> Map10 [order 1] : after(500,tick)
      | [BSteeringWheelButton5 ==1]
  data: rTorqueSplit output double; BSteeringWheelButton2 input boolean; BSteeringWheelButton5 input boolean

== stateflow chart SteeringWheel/DDU7 Display Number 5 System/PRegen System ==
  state Map12
    entry:
    PRegen = 10;
  state Map7
    entry, during:
    PRegen = 15;
  state Map8
    entry, during:
    PRegen = 20;
  state Map9
    entry, during:
    PRegen = 30;
  state Map10
    entry, during:
    PRegen = 40;
  state Map11
    entry, during:
    PRegen = 0;
  Map9 -> Map10 [order 2] : after(500,tick)
      | [BSteeringWheelButton2 == 1]
  Map8 -> Map9 [order 2] : after(500,tick)
      | [BSteeringWheelButton2 == 1]
  Map10 -> Map11 [order 2] : after(500,tick)
      | [BSteeringWheelButton2 == 1]
  Map7 -> Map8 [order 2] : after(500,tick)
      | [BSteeringWheelButton2 == 1]
  Map12 -> Map7 [order 1] : after(500,tick)
      | [BSteeringWheelButton2 == 1]
  (default) -> Map12
  Map12 -> Map11 [order 2] : after(500,tick)
      | [BSteeringWheelButton5 ==1]
  Map11 -> Map12 [order 2] : after(500,tick)
      | [BSteeringWheelButton2 == 1]
  Map7 -> Map12 [order 1] : after(500,tick)
      | [BSteeringWheelButton5 ==1]
  Map8 -> Map7 [order 1] : after(500,tick)
      | [BSteeringWheelButton5 ==1]
  Map9 -> Map8 [order 1] : after(500,tick)
      | [BSteeringWheelButton5 ==1]
  Map10 -> Map9 [order 1] : after(500,tick)
      | [BSteeringWheelButton5 ==1]
  Map11 -> Map10 [order 1] : after(500,tick)
      | [BSteeringWheelButton5 ==1]
  data: PRegen output double; BSteeringWheelButton2 input boolean; BSteeringWheelButton5 input boolean

== stateflow chart SteeringWheel/DDU7 Display Number 5 System/BSpinningModelActivated System ==
  state Map12
    entry:
    BSpinningModelActivated = 1;
  state Map11
    entry, during:
    BSpinningModelActivated = 0;
  Map11 -> Map12 [order 2] : after(500,tick)
      | [BSteeringWheelButton5 ==1]
  Map12 -> Map11 [order 2] : after(500,tick)
      | [BSteeringWheelButton2 == 1]
  (default) -> Map11
  Map12 -> Map11 [order 1] : after(500,tick)
      | [BSteeringWheelButton5 ==1]
  Map11 -> Map12 [order 1] : after(500,tick)
      | [BSteeringWheelButton2 == 1]
  data: BSpinningModelActivated output double; BSteeringWheelButton2 input boolean; BSteeringWheelButton5 input boolean

== stateflow chart SteeringWheel/DDU7 Display Number 5 System/NThrottleMap System ==
  state Map12
    entry:
    NThrottleMap = 1;
    PDischarge = 30;
  state Map7
    entry, during:
    NThrottleMap = 2;
    PDischarge = 45;
  state Map8
    entry, during:
    NThrottleMap = 3;
    PDischarge = 77;
  state Map9
    entry, during:
    NThrottleMap = 4;
    PDischarge = 40;
  state Map10
    entry, during:
    NThrottleMap = 5;
    PDischarge = 77;
  state Map13
    entry, during:
    NThrottleMap = 6;
    PDischarge = 58;
  Map8 -> Map9 [order 2] : after(500,tick)
      | [BSteeringWheelButton2 == 1]
  Map10 -> Map13 [order 2] : after(500,tick)
      | [BSteeringWheelButton2 == 1]
  Map9 -> Map10 [order 2] : after(500,tick)
      | [BSteeringWheelButton2 == 1]
  Map7 -> Map8 [order 2] : after(500,tick)
      | [BSteeringWheelButton2 == 1]
  Map12 -> Map7 [order 2] : after(500,tick)
      | [BSteeringWheelButton2 == 1]
  (default) -> Map12
  Map7 -> Map12 [order 1] : after(500,tick)
      | [BSteeringWheelButton5 ==1]
  Map8 -> Map7 [order 1] : after(500,tick)
      | [BSteeringWheelButton5 ==1]
  Map9 -> Map8 [order 1] : after(500,tick)
      | [BSteeringWheelButton5 ==1]
  Map10 -> Map9 [order 1] : after(500,tick)
      | [BSteeringWheelButton5 ==1]
  Map13 -> Map10 [order 1] : after(500,tick)
      | [BSteeringWheelButton5 ==1]
  Map12 -> Map13 [order 1] : after(500,tick)
      | [BSteeringWheelButton5 ==1]
  Map13 -> Map12 [order 2] : after(500,tick)
      | [BSteeringWheelButton2 == 1]
  data: NThrottleMap output double; BSteeringWheelButton2 input boolean; BSteeringWheelButton5 input boolean; PDischarge output double

== stateflow chart SteeringWheel/NModeNumber System/NModeNumberDisplay6 System ==
  state Reset10
    Reset=1;
  state Reset4
    Reset=1;
  state Reset
    Reset=1;
  state Reset1
    Reset=1;
  state Reset2
    Reset=1;
  state Reset3
    Reset=1;
  state Mode12
    entry:
    NModeNumberDisplay6 = 1;
    Reset =0;
  state Mode8
    entry, during:
    NModeNumberDisplay6 = 3;
    Reset =0;
  state Mode10
    entry, during:
    NModeNumberDisplay6 = 6;
    Reset =0;
  state Mode9
    entry, during:
    NModeNumberDisplay6 = 5;
    Reset =0;
  state Mode7
    entry, during:
    NModeNumberDisplay6 = 2;
    Reset =0;
  state Mode11
    entry, during:
    NModeNumberDisplay6 = 4;
    Reset =0;
  state Reset5
    Reset=1;
  state Reset8
    Reset=1;
  state Reset9
    Reset=1;
  state Reset7
    Reset=1;
  state Reset6
    Reset=1;
  state Reset11
    Reset=1;
  Reset10 -> Mode12 : after(50,tick)
  Mode10 -> Reset10 [order 2] : after(500,tick)
      | [BSteeringWheelButton4 == 1]
  Reset2 -> Mode11 : after(50,tick)
  Reset -> Mode7 : after(50,tick)
  Reset1 -> Mode8 : after(50,tick)
  Reset3 -> Mode9 : after(50,tick)
  Mode9 -> Reset4 [order 1] : after(500,tick)
      | [BSteeringWheelButton4 == 1]
  Reset4 -> Mode10 : after(50,tick)
  Mode11 -> Reset3 [order 1] : after(500,tick)
      | [BSteeringWheelButton4 == 1]
  Mode7 -> Reset1 [order 2] : after(500,tick)
      | [BSteeringWheelButton4 == 1]
  Mode8 -> Reset2 [order 2] : after(500,tick)
      | [BSteeringWheelButton4 == 1]
  Mode12 -> Reset [order 1] : after(500,tick)
      | [BSteeringWheelButton4 == 1]
  (default) -> Mode12
  Mode7 -> Reset9 [order 1] : after(500,tick)
      | [BSteeringWheelButton6 ==1]
  Reset8 -> Mode7 : after(50,tick)
  Mode8 -> Reset8 [order 1] : after(500,tick)
      | [BSteeringWheelButton6 ==1]
  Reset7 -> Mode8 : after(50,tick)
  Mode11 -> Reset7 [order 2] : after(500,tick)
      | [BSteeringWheelButton6 ==1]
  Reset6 -> Mode11 : after(50,tick)
  Mode9 -> Reset6 [order 2] : after(500,tick)
      | [BSteeringWheelButton6 ==1]
  Reset5 -> Mode9 : after(50,tick)
  Reset11 -> Mode10 : after(50,tick)
  Mode10 -> Reset5 [order 1] : after(500,tick)
      | [BSteeringWheelButton6 ==1]
  Mode12 -> Reset11 [order 2] : after(500,tick)
      | [BSteeringWheelButton6 ==1]
  Reset9 -> Mode12 : after(50,tick)
  data: BSteeringWheelButton4 input boolean; NModeNumberDisplay6 output; BSteeringWheelButton6 input boolean; Reset local

== stateflow chart SteeringWheel/DDU7 Display Number 6 System/BAccumulatorFanOn System ==
  state Map13
    entry:
    BAccumulatorFanOn = 0;
  state Map14
    entry, during:
    BAccumulatorFanOn = 1;
  Map14 -> Map13 [order 2] : after(500,tick)
      | [BSteeringWheelButton5 ==1]
  (default) -> Map13
  Map13 -> Map14 [order 2] : after(500,tick)
      | [BSteeringWheelButton2 == 1]
  Map13 -> Map14 [order 1] : after(500,tick)
      | [BSteeringWheelButton5 ==1]
  Map14 -> Map13 [order 1] : after(500,tick)
      | [BSteeringWheelButton2 == 1]
  data: BAccumulatorFanOn output double; BSteeringWheelButton2 input boolean; BSteeringWheelButton5 input boolean

== stateflow chart SteeringWheel/DDU7 Display Number 6 System/rTorqueVectoringMultiplier System ==
  state Map12
    entry:
    rTorqueVectoringMultiplier = 0.1;
  state Map7
    entry, during:
    rTorqueVectoringMultiplier = 0.3;
  state Map8
    entry, during:
    rTorqueVectoringMultiplier = 0.5;
  state Map9
    entry, during:
    rTorqueVectoringMultiplier = 0.7;
  state Map10
    entry, during:
    rTorqueVectoringMultiplier = 0.85;
  state Map11
    entry, during:
    rTorqueVectoringMultiplier = 1;
  (default) -> Map8
  Map8 -> Map9 [order 2] : after(500,tick)
      | [BSteeringWheelButton2 == 1]
  Map9 -> Map10 [order 2] : after(500,tick)
      | [BSteeringWheelButton2 == 1]
  Map10 -> Map11 [order 2] : after(500,tick)
      | [BSteeringWheelButton2 == 1]
  Map7 -> Map8 [order 2] : after(500,tick)
      | [BSteeringWheelButton2 == 1]
  Map12 -> Map7 [order 1] : after(500,tick)
      | [BSteeringWheelButton2 == 1]
  Map12 -> Map11 [order 2] : after(500,tick)
      | [BSteeringWheelButton5 ==1]
  Map11 -> Map12 [order 2] : after(500,tick)
      | [BSteeringWheelButton2 == 1]
  Map8 -> Map7 [order 1] : after(500,tick)
      | [BSteeringWheelButton5 ==1]
  Map9 -> Map8 [order 1] : after(500,tick)
      | [BSteeringWheelButton5 ==1]
  Map10 -> Map9 [order 1] : after(500,tick)
      | [BSteeringWheelButton5 ==1]
  Map11 -> Map10 [order 1] : after(500,tick)
      | [BSteeringWheelButton5 ==1]
  Map7 -> Map12 [order 1] : after(500,tick)
      | [BSteeringWheelButton5 ==1]
  data: rTorqueVectoringMultiplier output double; BSteeringWheelButton2 input boolean; BSteeringWheelButton5 input boolean

== stateflow chart SteeringWheel/DDU7 Display Number 6 System/NTorqueSplitSpeedSelector System ==
  state Map12
    entry:
    NTorqueSplitSpeedSelector = 1;
  state Map11
    entry, during:
    NTorqueSplitSpeedSelector = 2;
  Map11 -> Map12 [order 2] : after(500,tick)
      | [BSteeringWheelButton5 ==1]
  Map12 -> Map11 [order 2] : after(500,tick)
      | [BSteeringWheelButton2 == 1]
  (default) -> Map11
  Map12 -> Map11 [order 1] : after(500,tick)
      | [BSteeringWheelButton5 ==1]
  Map11 -> Map12 [order 1] : after(500,tick)
      | [BSteeringWheelButton2 == 1]
  data: BSteeringWheelButton2 input boolean; BSteeringWheelButton5 input boolean; NTorqueSplitSpeedSelector output

== stateflow chart SteeringWheel/DDU7 Display Number 6 System/NPowerControllerKpSelector System ==
  state Map9
    entry, during:
    NPowerControllerKpSelector = 4;
  state Map12
    entry:
    NPowerControllerKpSelector = 1;
  state Map7
    entry, during:
    NPowerControllerKpSelector = 2;
  state Map11
    entry, during:
    NPowerControllerKpSelector = 6;
  state Map10
    entry, during:
    NPowerControllerKpSelector = 5;
  state Map8
    entry, during:
    NPowerControllerKpSelector = 3;
  (default) -> Map8
  Map9 -> Map10 [order 2] : after(500,tick)
      | [BSteeringWheelButton2 == 1]
  Map8 -> Map9 [order 2] : after(500,tick)
      | [BSteeringWheelButton2 == 1]
  Map10 -> Map11 [order 2] : after(500,tick)
      | [BSteeringWheelButton2 == 1]
  Map7 -> Map8 [order 2] : after(500,tick)
      | [BSteeringWheelButton2 == 1]
  Map12 -> Map7 [order 1] : after(500,tick)
      | [BSteeringWheelButton2 == 1]
  Map12 -> Map11 [order 2] : after(500,tick)
      | [BSteeringWheelButton5 ==1]
  Map11 -> Map12 [order 2] : after(500,tick)
      | [BSteeringWheelButton2 == 1]
  Map7 -> Map12 [order 1] : after(500,tick)
      | [BSteeringWheelButton5 ==1]
  Map8 -> Map7 [order 1] : after(500,tick)
      | [BSteeringWheelButton5 ==1]
  Map9 -> Map8 [order 1] : after(500,tick)
      | [BSteeringWheelButton5 ==1]
  Map10 -> Map9 [order 1] : after(500,tick)
      | [BSteeringWheelButton5 ==1]
  Map11 -> Map10 [order 1] : after(500,tick)
      | [BSteeringWheelButton5 ==1]
  data: NPowerControllerKpSelector output double; BSteeringWheelButton2 input boolean; BSteeringWheelButton5 input boolean

== stateflow chart SteeringWheel/DDU7 Display Number 6 System/BTractionControlActivated System ==
  state Map12
    entry:
    BTractionControlActivated = 1;
  state Map11
    entry, during:
    BTractionControlActivated = 0;
  Map11 -> Map12 [order 2] : after(500,tick)
      | [BSteeringWheelButton5 ==1]
  Map12 -> Map11 [order 2] : after(500,tick)
      | [BSteeringWheelButton2 == 1]
  (default) -> Map11
  Map12 -> Map11 [order 1] : after(500,tick)
      | [BSteeringWheelButton5 ==1]
  Map11 -> Map12 [order 1] : after(500,tick)
      | [BSteeringWheelButton2 == 1]
  data: BTractionControlActivated output double; BSteeringWheelButton2 input boolean; BSteeringWheelButton5 input boolean

== stateflow chart SteeringWheel/DDU7 Display Number 6 System/NTractionControlKpSelector System ==
  state Map12
    entry:
    NTractionControlKpSelector = 1;
  state Map8
    entry, during:
    NTractionControlKpSelector = 3;
  state Map7
    entry, during:
    NTractionControlKpSelector = 2;
  state Map13
    entry, during:
    NTractionControlKpSelector = 4;
  Map7 -> Map8 [order 2] : after(500,tick)
      | [BSteeringWheelButton2 == 1]
  Map8 -> Map13 [order 2] : after(500,tick)
      | [BSteeringWheelButton2 == 1]
  Map12 -> Map7 [order 2] : after(500,tick)
      | [BSteeringWheelButton2 == 1]
  (default) -> Map7
  Map7 -> Map12 [order 1] : after(500,tick)
      | [BSteeringWheelButton5 ==1]
  Map8 -> Map7 [order 1] : after(500,tick)
      | [BSteeringWheelButton5 ==1]
  Map13 -> Map8 [order 2] : after(500,tick)
      | [BSteeringWheelButton5 ==1]
  Map12 -> Map13 [order 1] : after(500,tick)
      | [BSteeringWheelButton5 ==1]
  Map13 -> Map12 [order 1] : after(500,tick)
      | [BSteeringWheelButton2 == 1]
  data: NTractionControlKpSelector output double; BSteeringWheelButton2 input boolean; BSteeringWheelButton5 input boolean

== stateflow chart SteeringWheel/DDU7 Display Number 1 System/BTorqueVectoringActivated Syatem ==
  state Map12
    entry:
    BTorqueVectoringActivated = 1;
  state Map11
    entry, during:
    BTorqueVectoringActivated = 0;
  (default) -> Map11
  Map12 -> Map11 : after(500,tick)
      | [BSteeringWheelButton5 ==1]
  Map11 -> Map12 : after(500,tick)
      | [BSteeringWheelButton2 == 1]
  data: BTorqueVectoringActivated output; BSteeringWheelButton2 input boolean; BSteeringWheelButton5 input boolean
